simulink model "flatpoint"  (R2022a)
settings: Solver=VariableStepAuto  StartTime=0.0  StopTime=1000.0  RelTol=1e-3
settings Model: Creator=Natriya  LastModifiedBy=Natriya

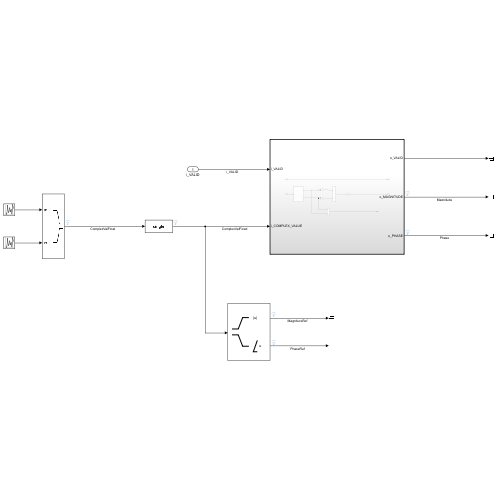
[thumbnail: Simulink's stored preview of the top-level diagram]
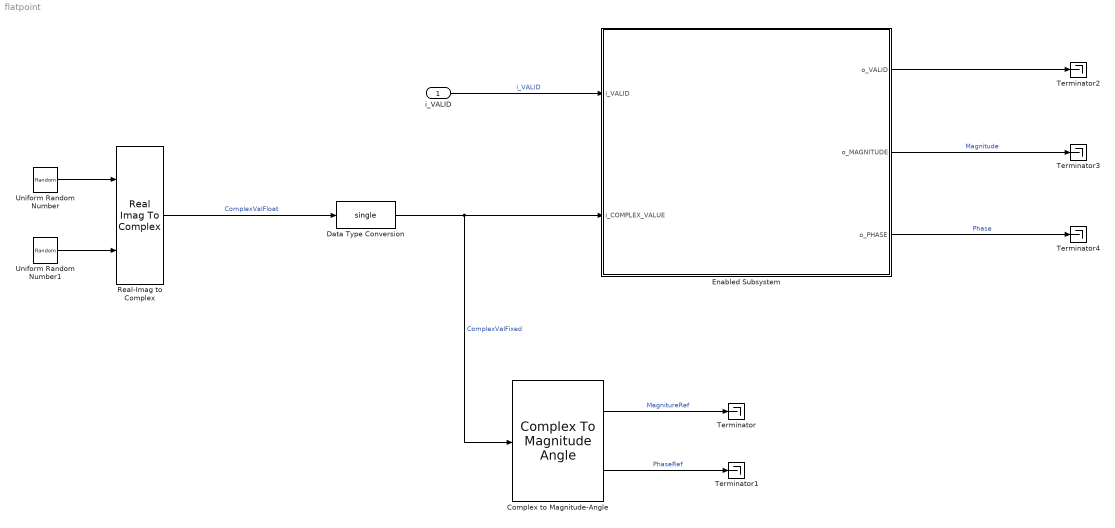
== system flatpoint ==
  i_VALID : Inport
  Complex to Magnitude-Angle : ComplexToMagnitudeAngle
  Data Type Conversion : DataTypeConversion  OutDataTypeStr=single  RndMeth=Round  SaturateOnIntegerOverflow=off
  Enabled Subsystem : Subsystem  TreatAsAtomicUnit=on
  Real-Imag to Complex : RealImagToComplex
  Terminator{,1..4} (5 alike) : Terminator
  Uniform Random Number : UniformRandomNumber  Minimum=-2^(23-1)  Maximum=2^(23-1)-1/2^9  Seed=23  SampleTime=1
  Uniform Random Number1 : UniformRandomNumber  Minimum=-2^(23-1)  Maximum=2^(23-1)-1/2^9  Seed=24  SampleTime=1
  wires:
  Enabled Subsystem/2(o_MAGNITUDE) -> Terminator3/1  "Magnitude"
  Data Type Conversion/1 -> Complex to Magnitude-Angle/1, Enabled Subsystem/2(i_COMPLEX_VALUE)  "ComplexValFixed"
  Complex to Magnitude-Angle/2 -> Terminator1/1  "PhaseRef"
  Enabled Subsystem/1(o_VALID) -> Terminator2/1
  Complex to Magnitude-Angle/1 -> Terminator/1  "MagnitureRef"
  Enabled Subsystem/3(o_PHASE) -> Terminator4/1  "Phase"
  Real-Imag to Complex/1 -> Data Type Conversion/1  "ComplexValFloat"
  Uniform Random Number1/1 -> Real-Imag to Complex/2
  i_VALID/1 -> Enabled Subsystem/1(i_VALID)  "i_VALID"
  Uniform Random Number/1 -> Real-Imag to Complex/1

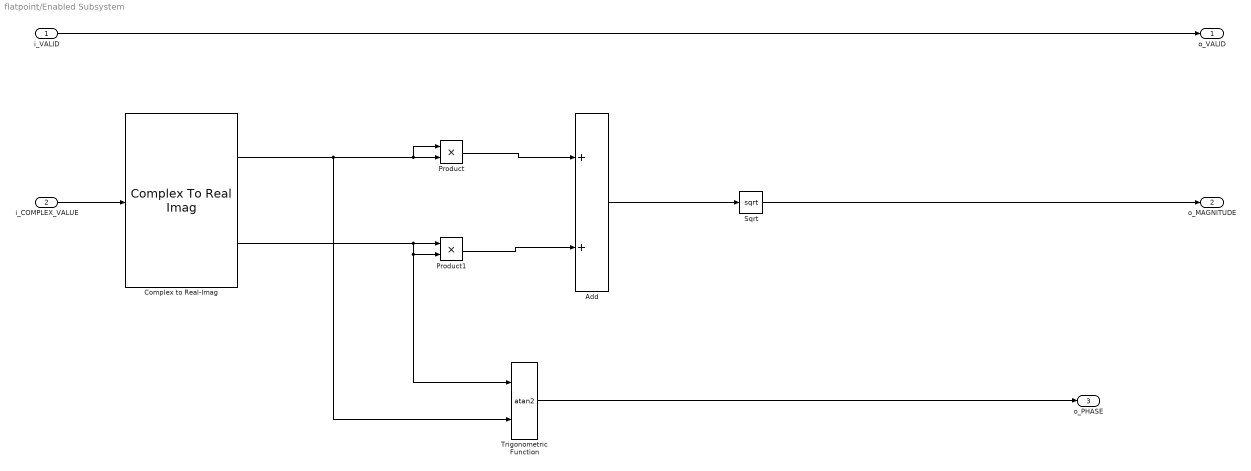
== system flatpoint/Enabled Subsystem ==
  i_VALID : Inport
  i_COMPLEX_VALUE : Inport  Port=2
  Add : Sum
  Complex to Real-Imag : ComplexToRealImag
  Product : Product
  Product1 : Product
  Sqrt : Sqrt  OutDataTypeStr=Inherit: Inherit via internal rule
  Trigonometric Function : Trigonometry  Operator=atan2
  o_VALID : Outport
  o_MAGNITUDE : Outport  Port=2  VectorParamsAs1DForOutWhenUnconnected=off
  o_PHASE : Outport  Port=3  VectorParamsAs1DForOutWhenUnconnected=off
  wires:
  i_VALID/1 -> o_VALID/1
  i_COMPLEX_VALUE/1 -> Complex to Real-Imag/1
  Complex to Real-Imag/1 -> Trigonometric Function/2, Product/1, Product/2
  Complex to Real-Imag/2 -> Product1/1, Trigonometric Function/1, Product1/2
  Product1/1 -> Add/2
  Product/1 -> Add/1
  Add/1 -> Sqrt/1
  Sqrt/1 -> o_MAGNITUDE/1
  Trigonometric Function/1 -> o_PHASE/1
